simulink model "PI_Controller0"  (R2020a)
settings: Solver=ode45  StartTime=0.0  StopTime=120  RelTol=1e-3
undefined symbols (not defined in the file): Ki, Kp
settings Model: DataDictionary=CruiseCtrl_data.sldd  Creator=NIKITA  LastModifiedBy=NIKITA
settings DataIOCC: SaveOutput=off  SaveTime=off

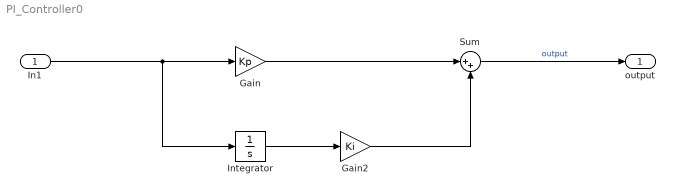
== system PI_Controller0 ==
  In1 : Inport  OutDataTypeStr=double  PortDimensions=1  SampleTime=0
  Gain : Gain  Gain=Kp
  Gain2 : Gain  Gain=Ki
  Integrator : Integrator
  Sum : Sum  Inputs=|++
  output : Outport  OutDataTypeStr=double  PortDimensions=1  SampleTime=0
  wires:
  Gain/1 -> Sum/1
  In1/1 -> Integrator/1, Gain/1
  Sum/1 -> output/1  "output"
  Integrator/1 -> Gain2/1
  Gain2/1 -> Sum/2
